simulink model "untitled"  (R2018b)
settings: Solver=ode3  StartTime=0.0  StopTime=10  RelTol=1e-3  EnableMultiTasking=on
libraries: arduinolib x4, arduinothingspeaklib x3, simulink x1
settings Model: FPTRunName=Active  ExtModeTrigDuration=2  Creator=Andrei  LastModifiedBy=Andrei
settings DataIOCC: LimitDataPoints=on  SaveFormat=Array
settings OptimizationCC: ExpressionDepthLimit=2147483647  LifeSpan=Inf  MaxStackSize=64
settings DebuggingCC: UnderspecifiedInitializationDetection=Classic  MergeDetectMultiDrivingBlocksExec=none  FcnCallInpInsideContextMsg=warning  AllowSymbolicDim=off  StateNameClashWarn=warning  SFUnexpectedBacktrackingDiag=warning  SFNoUnconditionalDefaultTransitionDiag=warning  SFExecutionAtInitializationDiag=none
settings HardwareCC: ProdBitPerInt=16  ProdBitPerPointer=16  ProdBitPerSizeT=16  ProdBitPerPtrDiffT=16  ProdLargestAtomicFloat=None  ProdWordSize=8  ProdHWDeviceType=Atmel->AVR  UseEmbeddedCoderFeatures=off  UseSimulinkCoderFeatures=off
settings ModelReferenceCC: PropagateSignalLabelsOutOfModel=off
settings SFSimCC: SimUseLocalCustomCode=off
settings RTWCC: SystemTargetFile=ert.tlc  HardwareBoard=Arduino Mega 2560  TemplateMakefile=ert_default_tmf  RTWVerbose=off  RTWUseLocalCustomCode=off  Toolchain=Arduino AVR  BuildConfiguration=Faster Runs
settings CodeAppCC: StateflowObjectComments=on
settings ERTTargetCC: MultiwordLength=2048  ERTCustomFileBanners=off  SupportContinuousTime=on  SupportNonInlinedSFcns=on  RemoveResetFunc=off  ModelStepFunctionPrototypeControlCompliant=off  ConvertIfToSwitch=off  SuppressUnreachableDefaultCases=off
settings ConfigComp: CovMetricSettings=dw  CovHtmlReporting=on  CovSaveCumulativeToWorkspaceVar=on  CovSaveSingleToWorkspaceVar=on  CovExternalEMLEnable=off  CovSFcnEnable=off

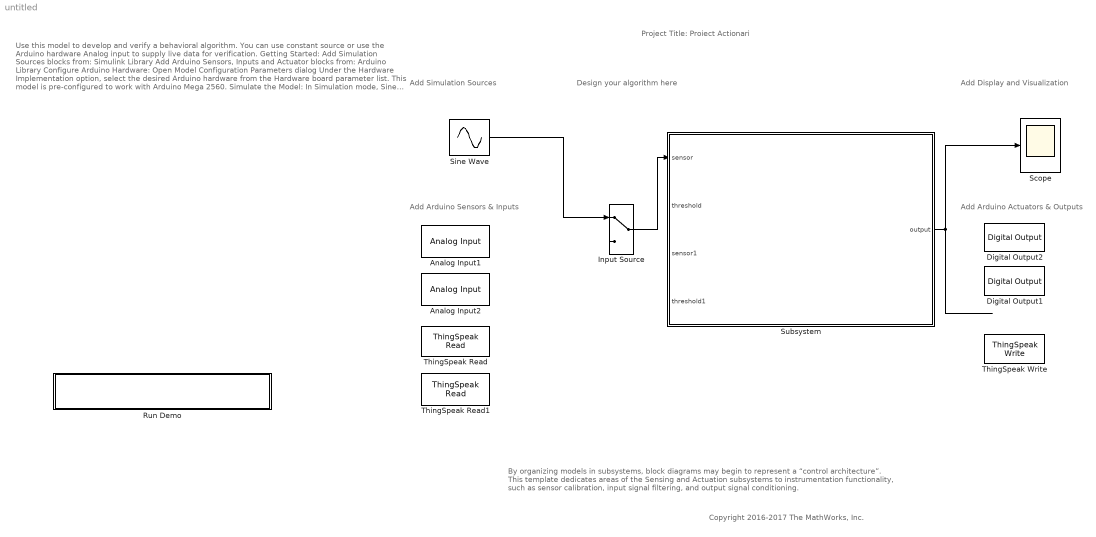
== system untitled ==
  note: Copyright 2016-2017 The MathWorks, Inc.
  note: Project Title: Proiect Actionari
  note: Use this model to develop and verify a behavioral algorithm. You can use constant source or use the Arduino hardware Analog input to supply live data for verification.
      |
      | Getting Started:
      |
      | Add Simulation Sources blocks from:
      | Simulink Library
      | Add Arduino Sensors, Inputs and Actuator blocks from:
      | Arduino Library
      |
      | Configure Arduino Hardware:
      |
      | Open Model Configuration Parameters dialog
      | Under the Hardware Implementation option, select the desired Arduino hardware from the Hardware board parameter list.
      | This model is pre-configured to work with Arduino Mega 2560.
      |
      | Simulate the Model:
      | In Simulation mode, Sine Wave Source block is used as an input to the algorithm and scope block to visualize the output data. During Simulation mode, Arduino Analog input and Digital ouput blocks does nothing.
      |
      | Double Click on the Input source switch in the model to select Sine Wave as the simulated input source for the algorithm.
      | Click Run on the Simulink Editor toolbar.
      |
      | Run the Model on Arduino Hardware (External Mode)
      |
      | Double click on the Input source switch in the model to select the sensor input as a source for the algorithm.
      | On the Simulink Editor toolbar, set Simulation mode to External .
      |
      | External mode will stop when the number of seconds specified in the Simulation stop time parameter elapses.
      |
      | Learn more:
      |
      | Simulink Subsystem
  note: Add Display and Visualization
  note: Add Arduino Sensors & Inputs
  note: Design your algorithm here
  note: Add Simulation Sources
  note: Add Arduino Actuators & Outputs
  note: By organizing models in subsystems, block diagrams may begin to represent a “control architecture”.
      | This template dedicates areas of the Sensing and Actuation subsystems to instrumentation functionality, such as sensor calibration, input signal filtering, and output signal conditioning.
  Analog Input1 : arduinolib/Analog Input  pinNumber=0  ReadResultsOnly=off  ConversionTriggerSource=Software  ExternalTriggerType=uint32(0)  OutputDataType=uint16  EnableConversionCompleteNotify=off  EnableOuputStatus=off  SampleTime=1  blockPlatform=arduino
  Analog Input2 : arduinolib/Analog Input  pinNumber=1  ReadResultsOnly=off  ConversionTriggerSource=Software  ExternalTriggerType=uint32(0)  OutputDataType=uint16  EnableConversionCompleteNotify=off  EnableOuputStatus=off  SampleTime=1  blockPlatform=arduino
  Digital Output1 : arduinolib/Digital Output  pinNumber=13  blockPlatform=arduino
  Digital Output2 : arduinolib/Digital Output  pinNumber=4  blockPlatform=arduino
  Input Source : ManualSwitch
  Run Demo : Subsystem  Description=Controls host-side RTDX processing.
      mask Display: pic=imread('arduinoExternalMode.png');image(pic);
  Scope : Scope
  Sine Wave : Sin  SineType=Sample based  Amplitude=1000  SampleTime=0.1
  Subsystem : Subsystem
  ThingSpeak Read : arduinothingspeaklib/ThingSpeak Read  ChannelID_=1049967  ChannelAccess_=Public  ReadAPIKey_=ABCDEFGHIJK  FieldNumber_=3  PrintDiagnosticMessages_=off  blockPlatform=Arduino  Interfacetype_=Ethernet  SampleTime_=60
      settings: SourceProductName=Simulink Support Package for Arduino Hardware  SourceProductBaseCode=ARDUINO
  ThingSpeak Read1 : arduinothingspeaklib/ThingSpeak Read  ChannelID_=1049967  ChannelAccess_=Public  ReadAPIKey_=ABCDEFGHIJK  FieldNumber_=4  PrintDiagnosticMessages_=off  blockPlatform=Arduino  Interfacetype_=Ethernet  SampleTime_=60
      settings: SourceProductName=Simulink Support Package for Arduino Hardware  SourceProductBaseCode=ARDUINO
  ThingSpeak Write : arduinothingspeaklib/ThingSpeak Write  ChannelID_=1049967  WriteAPIKey_=L9XOCJV3K8M5YF2W  NumberOfFields=2  UpdateInterval_=60  PrintDiagnosticMessages_=off  LocationEnabled=off  LocationSource=Block dialog  blockPlatform=arduino  Interfacetype_=Ethernet  UpdateURL=0  StatusMessage=0  StatusEnabled=on  StatusSource=<empty>
      settings: SourceProductName=Simulink Support Package for Arduino Hardware  SourceProductBaseCode=ARDUINO
  wires:
  Input Source/1 -> Subsystem/1(sensor)
  Sine Wave/1 -> Input Source/1
  ? -> Input Source/2
  Subsystem/1(output) -> Scope/1

== system untitled/Run Demo ==

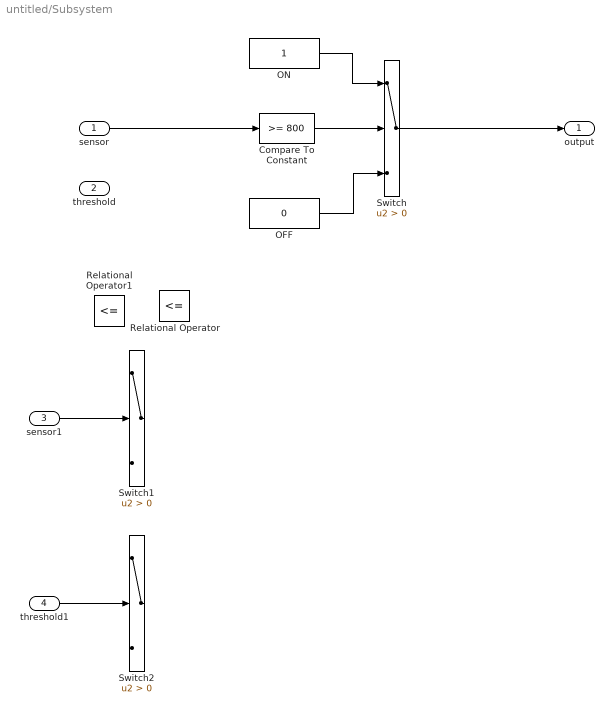
== system untitled/Subsystem ==
  sensor : Inport
  threshold : Inport  Port=2
  sensor1 : Inport  Port=3
  threshold1 : Inport  Port=4
  Compare To Constant : simulink/Logic and Bit Operations/Compare To Constant  relop=>=  const=800  OutDataTypeStr=boolean
  OFF : Constant  Value=0  SampleTime=-1
  ON : Constant  SampleTime=-1
  Relational Operator : RelationalOperator  Operator=<=  OutDataTypeStr=boolean  RndMeth=Simplest
  Relational Operator1 : RelationalOperator  Operator=<=  OutDataTypeStr=boolean  RndMeth=Simplest
  Switch : Switch  Criteria=u2 > Threshold
  Switch1 : Switch  Criteria=u2 > Threshold
  Switch2 : Switch  Criteria=u2 > Threshold
  output : Outport
  wires:
  Compare To Constant/1 -> Switch/2
  Switch/1 -> output/1
  sensor/1 -> Compare To Constant/1
  OFF/1 -> Switch/3
  ON/1 -> Switch/1
  sensor1/1 -> Switch1/2
  threshold1/1 -> Switch2/2
